simulink model "Traj_plt"  (R2023a)
settings: Solver=VariableStepAuto  StartTime=0.0  StopTime=inf  RelTol=1e-3
values from neighbouring files (symbols this model uses):
  beta = beta_i'.*task    [Compare1.m]    (also in Compare2.m; Final1.m; Final2.m; Final3.m)
undefined symbols (not defined in the file or in its folder): B_prev, Bst, Bst_prev, convertStringsToChars, dist_C, DroneMass, Earth, Gravity, h_ref, initialState, quad_pos, sinit, stack_size, task_mat, WGS84
libraries: slpidlib x66, aerolibconvert2 x11, aerolibtransform2 x11, uavalgslib x11, dspsrcs4 x1
(part 2 of 12)

== system Traj_plt/agent_4/Quad_1/Inner Loop and Plant Model ==
  PositionCmds : Inport
  Low-FidelityModel : Subsystem  VariantControl=plantModelFi ==0
  Out1 : Outport

== system Traj_plt/agent_5/Quad_1/Inner Loop and Plant Model ==
  PositionCmds : Inport
  Low-FidelityModel : Subsystem  VariantControl=plantModelFi ==0
  Out1 : Outport

== system Traj_plt/agent_6/Quad_1/Inner Loop and Plant Model ==
  PositionCmds : Inport
  Low-FidelityModel : Subsystem  VariantControl=plantModelFi ==0
  Out1 : Outport

== system Traj_plt/agent_7/Quad_1/Inner Loop and Plant Model ==
  PositionCmds : Inport
  Low-FidelityModel : Subsystem  VariantControl=plantModelFi ==0
  Out1 : Outport

== system Traj_plt/agent_8/Quad_1/Inner Loop and Plant Model ==
  PositionCmds : Inport
  Low-FidelityModel : Subsystem  VariantControl=plantModelFi ==0
  Out1 : Outport

== system Traj_plt/agent_9/Quad_1/Inner Loop and Plant Model ==
  PositionCmds : Inport
  Low-FidelityModel : Subsystem  VariantControl=plantModelFi ==0
  Out1 : Outport

== system Traj_plt/agent_1/Quad_1/Inner Loop and Plant Model/Low-FidelityModel ==
  PositionCmds : Inport
  Assemble UAV State Bus : Subsystem
  Bus Creator : BusCreator  Inputs=1
  Bus Creator1 : BusCreator  Inputs=1  OutDataTypeStr=Bus: uavGuidanceEnvironmentBus  NonVirtualBus=on
  Constant : Constant  Value=9.8  OutDataTypeStr=single
      settings: AttributesFormatString=%<Value>
  Position and Acceleration Control : Subsystem
  Quadrotor Plant : Subsystem  AncestorBlock=uavalgslib/Guidance Model  mask(Guidance Model){ModelType=MultirotorGuidance, SpecifiedDataType=single, SimulateUsing=Code generation, InitialWorldPositionMultirotor=quad_pos(:,1), InitialWorldVelocityMultirotor=[0; 0; 0], InitialEulerZYXMultirotor=[0; 0; 0], InitialBodyAngularRateRPYMultirotor=[0; 0; 0], InitialThrustMultirotor=0, InitialNorthFixedWing=0, InitialEastFixedWing=0, InitialHeightFixedWing=0, InitialAirSpeedFixedWing=0, InitialHeadingAngleFixedWing=0, InitialFlightPathAngleFixedWing=0, InitialRollAngleFixedWing=0, InitialRollAngleRateFixedWing=0, PDRollMultirotor=[3402.97,116.67], PDPitchMultirotor=[3402.97, 116.67], PYawRateMultirotor=1950, PThrustMultirotor=39, MassMultirotor=0.1, PHeightFixedWing=3.9, PHeadingAngleFixedWing=3.9, PFlightPathAngleFixedWing=39, PDRollFixedWing=[3402.97, 116.67], PAirSpeedFixedWing=1, FlightPathAngleLimitsFixedWing=[-pi/2, pi/2], StateBusName='uavGuidanceStateBus', ControlBusName='uavGuidanceControlBus', EnvironmentBusName='uavGuidanceEnvironmentBus', DataType=single}
      mask prompts: ModelType "uav:robotsluav:guidancemodelblock:ModelType"; SpecifiedDataType "uav:robotsluav:guidancemodelblock:DataType"; SimulateUsing "SystemBlock:MATLABSystem:SimulateUsing"; InitialWorldPositionMultirotor "uav:robotsluav:guidancemodelblock:WorldPosition"; InitialWorldVelocityMultirotor "uav:robotsluav:guidancemodelblock:WorldVelocity"; InitialEulerZYXMultirotor "uav:robotsluav:guidancemodelblock:EulerZYX"; InitialBodyAngularRateRPYMultirotor "uav:robotsluav:guidancemodelblock:BodyAngularRateRPY"; InitialThrustMultirotor "uav:robotsluav:guidancemodelblock:Thrust"; InitialNorthFixedWing "uav:robotsluav:guidancemodelblock:NorthPosition"; InitialEastFixedWing "uav:robotsluav:guidancemodelblock:EastPosition"; InitialHeightFixedWing "uav:robotsluav:guidancemodelblock:Height"; InitialAirSpeedFixedWing "uav:robotsluav:guidancemodelblock:AirSpeed"; InitialHeadingAngleFixedWing "uav:robotsluav:guidancemodelblock:HeadingAngle"; InitialFlightPathAngleFixedWing "uav:robotsluav:guidancemodelblock:FlightPathAngle"; InitialRollAngleFixedWing "uav:robotsluav:guidancemodelblock:RollAngle"; InitialRollAngleRateFixedWing "uav:robotsluav:guidancemodelblock:RollAngleRate"; PDRollMultirotor "uav:robotsluav:guidancemodelblock:PDRoll"; PDPitchMultirotor "uav:robotsluav:guidancemodelblock:PDPitch"; PYawRateMultirotor "uav:robotsluav:guidancemodelblock:PYawRate"; PThrustMultirotor "uav:robotsluav:guidancemodelblock:PThrust"; MassMultirotor "uav:robotsluav:guidancemodelblock:Mass"; PHeightFixedWing "uav:robotsluav:guidancemodelblock:PHeight"; PHeadingAngleFixedWing "uav:robotsluav:guidancemodelblock:PHeadingAngle"; PFlightPathAngleFixedWing "uav:robotsluav:guidancemodelblock:PFlightPathAngle"; PDRollFixedWing "uav:robotsluav:guidancemodelblock:PDRollAngle"; PAirSpeedFixedWing "uav:robotsluav:guidancemodelblock:PAirSpeed"; FlightPathAngleLimitsFixedWing "uav:robotsluav:guidancemodelblock:MinMaxFlightPathAngle"; StateBusName "uav:robotsluav:guidancemodelblock:StateBusName"; ControlBusName "uav:robotsluav:guidancemodelblock:ControlBusName"; EnvironmentBusName "uav:robotsluav:guidancemodelblock:EnvironmentBusName"; DataType "uav:robotsluav:guidancemodelblock:ResolvedDataType"
      mask help: uav:robotsluav:guidancemodelblock:Description
      mask init:
      | ModelName = gcb;
      | 
      | % Validate bus names
      | uav.sluav.internal.guidancemodel.mask.validateBusNames(gcb);
      | 
      | [stateDimension, initialState, UAVType, UAVDataType, UAVConfig] = ...
      |     uav.sluav.internal.guidancemodel.mask.initialize(ModelName, ModelType, gcb);
      mask Help: eval('helpview(fullfile(docroot, ''uav'', ''helptargets.map''), ''uavGuidanceModelBlock'')');
      mask TypeOptions ModelType: uav:robotsluav:guidancemodelblock:ModelTypeMultirotor | uav:robotsluav:guidancemodelblock:ModelTypeFixedWing
      mask Callback ModelType:
      | % Change mask dialog
      | uav.sluav.internal.guidancemodel.mask.modelTypeCallback(gcb);
      | 
      | % Create buses for the UAV block
      | uav.sluav.internal.guidancemodel.mask.createUAVBuses(gcb);
      mask Callback SpecifiedDataType:
      | if ~strcmp(get_param(gcb, 'SpecifiedDataType'), '<data type expression>')
      |     % Resolve input type
      |     uav.sluav.internal.guidancemodel.mask.dataTypeCallback(gcb);
      | 
      |     % Create buses for the UAV block
      |     uav.sluav.internal.guidancemodel.mask.createUAVBuses(gcb);
      | end
      mask TypeOptions SimulateUsing: ComputeDerivative/SimulateUsing | StateVector2Struct/SimulateUsing
      mask Callback StateBusName:
      | % Validate bus names
      | uav.sluav.internal.guidancemodel.mask.validateBusNames(gcb);
      | 
      | % Create buses for the UAV block
      | uav.sluav.internal.guidancemodel.mask.createUAVBuses(gcb);
      mask Callback ControlBusName:
      | % Validate bus names
      | uav.sluav.internal.guidancemodel.mask.validateBusNames(gcb);
      | 
      | % Create buses for the UAV block
      | uav.sluav.internal.guidancemodel.mask.createUAVBuses(gcb);
      mask Callback EnvironmentBusName:
      | % Validate bus names
      | uav.sluav.internal.guidancemodel.mask.validateBusNames(gcb);
      | 
      | % Create buses for the UAV block
      | uav.sluav.internal.guidancemodel.mask.createUAVBuses(gcb);
      mask DialogControl ModelType Prompt: Model Type:
      mask DialogControl SpecifiedDataType Prompt: Data Type:
      mask DialogControl SimulateUsing Prompt: Simulate using:
      mask DialogControl SimulateUsing Tooltip: SystemBlock:MATLABSystem:SimulateUsingDescription
      mask DialogControl InitialStateTab Prompt: uav:robotsluav:guidancemodelblock:InitialState
      mask DialogControl InitialWorldPositionMultirotor Prompt: World Position
      mask DialogControl InitialWorldVelocityMultirotor Prompt: World Velocity
      mask DialogControl InitialEulerZYXMultirotor Prompt: Euler Angles (ZYX)
      mask DialogControl InitialBodyAngularRateRPYMultirotor Prompt: Body Angular Rate
      mask DialogControl InitialThrustMultirotor Prompt: Thrust
      mask DialogControl InitialNorthFixedWing Prompt: North Position
      mask DialogControl InitialEastFixedWing Prompt: East Position
      mask DialogControl InitialHeightFixedWing Prompt: Height
      mask DialogControl InitialAirSpeedFixedWing Prompt: Air Speed
      mask DialogControl InitialHeadingAngleFixedWing Prompt: Heading Angle
      mask DialogControl InitialFlightPathAngleFixedWing Prompt: Flight Path Angle
      mask DialogControl InitialRollAngleFixedWing Prompt: Roll Angle
      mask DialogControl InitialRollAngleRateFixedWing Prompt: Roll Angular Velocity
      mask DialogControl ConfigurationTab Prompt: uav:robotsluav:guidancemodelblock:Configuration
      mask DialogControl PDRollMultirotor Prompt: PD Roll
      mask DialogControl PDPitchMultirotor Prompt: PD Pitch
      mask DialogControl PYawRateMultirotor Prompt: P YawRate
      mask DialogControl PThrustMultirotor Prompt: P Thrust
      mask DialogControl MassMultirotor Prompt: Mass
      mask DialogControl PHeightFixedWing Prompt: P Height
      mask DialogControl PHeadingAngleFixedWing Prompt: P Heading Angle
      mask DialogControl PFlightPathAngleFixedWing Prompt: P Flight Path Angle
      mask DialogControl PDRollFixedWing Prompt: PD Roll Angle
      mask DialogControl PAirSpeedFixedWing Prompt: P Air Speed
      mask DialogControl FlightPathAngleLimitsFixedWing Prompt: Min/Max Flight Path Angle
      mask DialogControl BusNameTab Prompt: uav:robotsluav:guidancemodelblock:InputOutputBusNames
      mask DialogControl StateBusName Prompt: State Bus Name
      mask DialogControl ControlBusName Prompt: Control Bus Name
      mask DialogControl EnvironmentBusName Prompt: Environment Bus Name
      mask DialogControl DataType Prompt: Resolved Data Type
      mask Display:
      | port_label('input', 1, 'Control')
      | port_label('input', 2, 'Environment')
      | port_label('output', 1, 'State')
  Rate Transition1 : RateTransition  OutPortSampleTime=UAVSampleTime
  Rate Transition2 : RateTransition  OutPortSampleTime=UAVSampleTime
  Out1 : Outport
  wires:
  Constant/1 -> Bus Creator1/1  "Gravity"
  Bus Creator1/1 -> Quadrotor Plant/2(Environment)
  Position and Acceleration Control/1(Control Signal) -> Rate Transition2/1
  Quadrotor Plant/1(State) -> Rate Transition1/1
  Rate Transition2/1 -> Quadrotor Plant/1(Control)
  PositionCmds/1 -> Position and Acceleration Control/2(PositionCmd)
  Rate Transition1/1 -> Position and Acceleration Control/1(QuadRotorState), Assemble UAV State Bus/1(State)
  Bus Creator/1 -> Out1/1
  Assemble UAV State Bus/1(UAVState) -> Bus Creator/1

== system Traj_plt/agent_10/Quad_1/Inner Loop and Plant Model/Low-FidelityModel ==
  PositionCmds : Inport
  Assemble UAV State Bus : Subsystem
  Bus Creator : BusCreator  Inputs=1
  Bus Creator1 : BusCreator  Inputs=1  OutDataTypeStr=Bus: uavGuidanceEnvironmentBus  NonVirtualBus=on
  Constant : Constant  Value=9.8  OutDataTypeStr=single
      settings: AttributesFormatString=%<Value>
  Position and Acceleration Control : Subsystem
  Quadrotor Plant : Subsystem  AncestorBlock=uavalgslib/Guidance Model  mask(Guidance Model){ModelType=MultirotorGuidance, SpecifiedDataType=single, SimulateUsing=Code generation, InitialWorldPositionMultirotor=quad_pos(:,10), InitialWorldVelocityMultirotor=[0; 0; 0], InitialEulerZYXMultirotor=[0; 0; 0], InitialBodyAngularRateRPYMultirotor=[0; 0; 0], InitialThrustMultirotor=0, InitialNorthFixedWing=0, InitialEastFixedWing=0, InitialHeightFixedWing=0, InitialAirSpeedFixedWing=0, InitialHeadingAngleFixedWing=0, InitialFlightPathAngleFixedWing=0, InitialRollAngleFixedWing=0, InitialRollAngleRateFixedWing=0, PDRollMultirotor=[3402.97,116.67], PDPitchMultirotor=[3402.97, 116.67], PYawRateMultirotor=1950, PThrustMultirotor=39, MassMultirotor=0.1, PHeightFixedWing=3.9, PHeadingAngleFixedWing=3.9, PFlightPathAngleFixedWing=39, PDRollFixedWing=[3402.97, 116.67], PAirSpeedFixedWing=1, FlightPathAngleLimitsFixedWing=[-pi/2, pi/2], StateBusName='uavGuidanceStateBus', ControlBusName='uavGuidanceControlBus', EnvironmentBusName='uavGuidanceEnvironmentBus', DataType=single}
      mask prompts: ModelType "uav:robotsluav:guidancemodelblock:ModelType"; SpecifiedDataType "uav:robotsluav:guidancemodelblock:DataType"; SimulateUsing "SystemBlock:MATLABSystem:SimulateUsing"; InitialWorldPositionMultirotor "uav:robotsluav:guidancemodelblock:WorldPosition"; InitialWorldVelocityMultirotor "uav:robotsluav:guidancemodelblock:WorldVelocity"; InitialEulerZYXMultirotor "uav:robotsluav:guidancemodelblock:EulerZYX"; InitialBodyAngularRateRPYMultirotor "uav:robotsluav:guidancemodelblock:BodyAngularRateRPY"; InitialThrustMultirotor "uav:robotsluav:guidancemodelblock:Thrust"; InitialNorthFixedWing "uav:robotsluav:guidancemodelblock:NorthPosition"; InitialEastFixedWing "uav:robotsluav:guidancemodelblock:EastPosition"; InitialHeightFixedWing "uav:robotsluav:guidancemodelblock:Height"; InitialAirSpeedFixedWing "uav:robotsluav:guidancemodelblock:AirSpeed"; InitialHeadingAngleFixedWing "uav:robotsluav:guidancemodelblock:HeadingAngle"; InitialFlightPathAngleFixedWing "uav:robotsluav:guidancemodelblock:FlightPathAngle"; InitialRollAngleFixedWing "uav:robotsluav:guidancemodelblock:RollAngle"; InitialRollAngleRateFixedWing "uav:robotsluav:guidancemodelblock:RollAngleRate"; PDRollMultirotor "uav:robotsluav:guidancemodelblock:PDRoll"; PDPitchMultirotor "uav:robotsluav:guidancemodelblock:PDPitch"; PYawRateMultirotor "uav:robotsluav:guidancemodelblock:PYawRate"; PThrustMultirotor "uav:robotsluav:guidancemodelblock:PThrust"; MassMultirotor "uav:robotsluav:guidancemodelblock:Mass"; PHeightFixedWing "uav:robotsluav:guidancemodelblock:PHeight"; PHeadingAngleFixedWing "uav:robotsluav:guidancemodelblock:PHeadingAngle"; PFlightPathAngleFixedWing "uav:robotsluav:guidancemodelblock:PFlightPathAngle"; PDRollFixedWing "uav:robotsluav:guidancemodelblock:PDRollAngle"; PAirSpeedFixedWing "uav:robotsluav:guidancemodelblock:PAirSpeed"; FlightPathAngleLimitsFixedWing "uav:robotsluav:guidancemodelblock:MinMaxFlightPathAngle"; StateBusName "uav:robotsluav:guidancemodelblock:StateBusName"; ControlBusName "uav:robotsluav:guidancemodelblock:ControlBusName"; EnvironmentBusName "uav:robotsluav:guidancemodelblock:EnvironmentBusName"; DataType "uav:robotsluav:guidancemodelblock:ResolvedDataType"
      mask help: uav:robotsluav:guidancemodelblock:Description
      mask init: same as Traj_plt/agent_1/Quad_1/Inner Loop and Plant Model/Low-FidelityModel/Quadrotor Plant
      mask Help: eval('helpview(fullfile(docroot, ''uav'', ''helptargets.map''), ''uavGuidanceModelBlock'')');
      mask TypeOptions ModelType: uav:robotsluav:guidancemodelblock:ModelTypeMultirotor | uav:robotsluav:guidancemodelblock:ModelTypeFixedWing
      mask Callback ModelType:
      | % Change mask dialog
      | uav.sluav.internal.guidancemodel.mask.modelTypeCallback(gcb);
      | 
      | % Create buses for the UAV block
      | uav.sluav.internal.guidancemodel.mask.createUAVBuses(gcb);
      mask Callback SpecifiedDataType:
      | if ~strcmp(get_param(gcb, 'SpecifiedDataType'), '<data type expression>')
      |     % Resolve input type
      |     uav.sluav.internal.guidancemodel.mask.dataTypeCallback(gcb);
      | 
      |     % Create buses for the UAV block
      |     uav.sluav.internal.guidancemodel.mask.createUAVBuses(gcb);
      | end
      mask TypeOptions SimulateUsing: ComputeDerivative/SimulateUsing | StateVector2Struct/SimulateUsing
      mask Callback StateBusName:
      | % Validate bus names
      | uav.sluav.internal.guidancemodel.mask.validateBusNames(gcb);
      | 
      | % Create buses for the UAV block
      | uav.sluav.internal.guidancemodel.mask.createUAVBuses(gcb);
      mask Callback ControlBusName:
      | % Validate bus names
      | uav.sluav.internal.guidancemodel.mask.validateBusNames(gcb);
      | 
      | % Create buses for the UAV block
      | uav.sluav.internal.guidancemodel.mask.createUAVBuses(gcb);
      mask Callback EnvironmentBusName:
      | % Validate bus names
      | uav.sluav.internal.guidancemodel.mask.validateBusNames(gcb);
      | 
      | % Create buses for the UAV block
      | uav.sluav.internal.guidancemodel.mask.createUAVBuses(gcb);
      mask DialogControl ModelType Prompt: Model Type:
      mask DialogControl SpecifiedDataType Prompt: Data Type:
      mask DialogControl SimulateUsing Prompt: Simulate using:
      mask DialogControl SimulateUsing Tooltip: SystemBlock:MATLABSystem:SimulateUsingDescription
      mask DialogControl InitialStateTab Prompt: uav:robotsluav:guidancemodelblock:InitialState
      mask DialogControl InitialWorldPositionMultirotor Prompt: World Position
      mask DialogControl InitialWorldVelocityMultirotor Prompt: World Velocity
      mask DialogControl InitialEulerZYXMultirotor Prompt: Euler Angles (ZYX)
      mask DialogControl InitialBodyAngularRateRPYMultirotor Prompt: Body Angular Rate
      mask DialogControl InitialThrustMultirotor Prompt: Thrust
      mask DialogControl InitialNorthFixedWing Prompt: North Position
      mask DialogControl InitialEastFixedWing Prompt: East Position
      mask DialogControl InitialHeightFixedWing Prompt: Height
      mask DialogControl InitialAirSpeedFixedWing Prompt: Air Speed
      mask DialogControl InitialHeadingAngleFixedWing Prompt: Heading Angle
      mask DialogControl InitialFlightPathAngleFixedWing Prompt: Flight Path Angle
      mask DialogControl InitialRollAngleFixedWing Prompt: Roll Angle
      mask DialogControl InitialRollAngleRateFixedWing Prompt: Roll Angular Velocity
      mask DialogControl ConfigurationTab Prompt: uav:robotsluav:guidancemodelblock:Configuration
      mask DialogControl PDRollMultirotor Prompt: PD Roll
      mask DialogControl PDPitchMultirotor Prompt: PD Pitch
      mask DialogControl PYawRateMultirotor Prompt: P YawRate
      mask DialogControl PThrustMultirotor Prompt: P Thrust
      mask DialogControl MassMultirotor Prompt: Mass
      mask DialogControl PHeightFixedWing Prompt: P Height
      mask DialogControl PHeadingAngleFixedWing Prompt: P Heading Angle
      mask DialogControl PFlightPathAngleFixedWing Prompt: P Flight Path Angle
      mask DialogControl PDRollFixedWing Prompt: PD Roll Angle
      mask DialogControl PAirSpeedFixedWing Prompt: P Air Speed
      mask DialogControl FlightPathAngleLimitsFixedWing Prompt: Min/Max Flight Path Angle
      mask DialogControl BusNameTab Prompt: uav:robotsluav:guidancemodelblock:InputOutputBusNames
      mask DialogControl StateBusName Prompt: State Bus Name
      mask DialogControl ControlBusName Prompt: Control Bus Name
      mask DialogControl EnvironmentBusName Prompt: Environment Bus Name
      mask DialogControl DataType Prompt: Resolved Data Type
      mask Display:
      | port_label('input', 1, 'Control')
      | port_label('input', 2, 'Environment')
      | port_label('output', 1, 'State')
  Rate Transition1 : RateTransition  OutPortSampleTime=UAVSampleTime
  Rate Transition2 : RateTransition  OutPortSampleTime=UAVSampleTime
  Out1 : Outport
  wires:
  Constant/1 -> Bus Creator1/1  "Gravity"
  Bus Creator1/1 -> Quadrotor Plant/2(Environment)
  Position and Acceleration Control/1(Control Signal) -> Rate Transition2/1
  Quadrotor Plant/1(State) -> Rate Transition1/1
  Rate Transition2/1 -> Quadrotor Plant/1(Control)
  PositionCmds/1 -> Position and Acceleration Control/2(PositionCmd)
  Rate Transition1/1 -> Position and Acceleration Control/1(QuadRotorState), Assemble UAV State Bus/1(State)
  Bus Creator/1 -> Out1/1
  Assemble UAV State Bus/1(UAVState) -> Bus Creator/1

== system Traj_plt/agent_11/Quad_1/Inner Loop and Plant Model/Low-FidelityModel ==
  PositionCmds : Inport
  Assemble UAV State Bus : Subsystem
  Bus Creator : BusCreator  Inputs=1
  Bus Creator1 : BusCreator  Inputs=1  OutDataTypeStr=Bus: uavGuidanceEnvironmentBus  NonVirtualBus=on
  Constant : Constant  Value=9.8  OutDataTypeStr=single
      settings: AttributesFormatString=%<Value>
  Position and Acceleration Control : Subsystem
  Quadrotor Plant : Subsystem  AncestorBlock=uavalgslib/Guidance Model  mask(Guidance Model){ModelType=MultirotorGuidance, SpecifiedDataType=single, SimulateUsing=Code generation, InitialWorldPositionMultirotor=quad_pos(:,6), InitialWorldVelocityMultirotor=[0; 0; 0], InitialEulerZYXMultirotor=[0; 0; 0], InitialBodyAngularRateRPYMultirotor=[0; 0; 0], InitialThrustMultirotor=0, InitialNorthFixedWing=0, InitialEastFixedWing=0, InitialHeightFixedWing=0, InitialAirSpeedFixedWing=0, InitialHeadingAngleFixedWing=0, InitialFlightPathAngleFixedWing=0, InitialRollAngleFixedWing=0, InitialRollAngleRateFixedWing=0, PDRollMultirotor=[3402.97,116.67], PDPitchMultirotor=[3402.97, 116.67], PYawRateMultirotor=1950, PThrustMultirotor=39, MassMultirotor=0.1, PHeightFixedWing=3.9, PHeadingAngleFixedWing=3.9, PFlightPathAngleFixedWing=39, PDRollFixedWing=[3402.97, 116.67], PAirSpeedFixedWing=1, FlightPathAngleLimitsFixedWing=[-pi/2, pi/2], StateBusName='uavGuidanceStateBus', ControlBusName='uavGuidanceControlBus', EnvironmentBusName='uavGuidanceEnvironmentBus', DataType=single}
      mask prompts: ModelType "uav:robotsluav:guidancemodelblock:ModelType"; SpecifiedDataType "uav:robotsluav:guidancemodelblock:DataType"; SimulateUsing "SystemBlock:MATLABSystem:SimulateUsing"; InitialWorldPositionMultirotor "uav:robotsluav:guidancemodelblock:WorldPosition"; InitialWorldVelocityMultirotor "uav:robotsluav:guidancemodelblock:WorldVelocity"; InitialEulerZYXMultirotor "uav:robotsluav:guidancemodelblock:EulerZYX"; InitialBodyAngularRateRPYMultirotor "uav:robotsluav:guidancemodelblock:BodyAngularRateRPY"; InitialThrustMultirotor "uav:robotsluav:guidancemodelblock:Thrust"; InitialNorthFixedWing "uav:robotsluav:guidancemodelblock:NorthPosition"; InitialEastFixedWing "uav:robotsluav:guidancemodelblock:EastPosition"; InitialHeightFixedWing "uav:robotsluav:guidancemodelblock:Height"; InitialAirSpeedFixedWing "uav:robotsluav:guidancemodelblock:AirSpeed"; InitialHeadingAngleFixedWing "uav:robotsluav:guidancemodelblock:HeadingAngle"; InitialFlightPathAngleFixedWing "uav:robotsluav:guidancemodelblock:FlightPathAngle"; InitialRollAngleFixedWing "uav:robotsluav:guidancemodelblock:RollAngle"; InitialRollAngleRateFixedWing "uav:robotsluav:guidancemodelblock:RollAngleRate"; PDRollMultirotor "uav:robotsluav:guidancemodelblock:PDRoll"; PDPitchMultirotor "uav:robotsluav:guidancemodelblock:PDPitch"; PYawRateMultirotor "uav:robotsluav:guidancemodelblock:PYawRate"; PThrustMultirotor "uav:robotsluav:guidancemodelblock:PThrust"; MassMultirotor "uav:robotsluav:guidancemodelblock:Mass"; PHeightFixedWing "uav:robotsluav:guidancemodelblock:PHeight"; PHeadingAngleFixedWing "uav:robotsluav:guidancemodelblock:PHeadingAngle"; PFlightPathAngleFixedWing "uav:robotsluav:guidancemodelblock:PFlightPathAngle"; PDRollFixedWing "uav:robotsluav:guidancemodelblock:PDRollAngle"; PAirSpeedFixedWing "uav:robotsluav:guidancemodelblock:PAirSpeed"; FlightPathAngleLimitsFixedWing "uav:robotsluav:guidancemodelblock:MinMaxFlightPathAngle"; StateBusName "uav:robotsluav:guidancemodelblock:StateBusName"; ControlBusName "uav:robotsluav:guidancemodelblock:ControlBusName"; EnvironmentBusName "uav:robotsluav:guidancemodelblock:EnvironmentBusName"; DataType "uav:robotsluav:guidancemodelblock:ResolvedDataType"
      mask help: uav:robotsluav:guidancemodelblock:Description
      mask init: same as Traj_plt/agent_1/Quad_1/Inner Loop and Plant Model/Low-FidelityModel/Quadrotor Plant
      mask Help: eval('helpview(fullfile(docroot, ''uav'', ''helptargets.map''), ''uavGuidanceModelBlock'')');
      mask TypeOptions ModelType: uav:robotsluav:guidancemodelblock:ModelTypeMultirotor | uav:robotsluav:guidancemodelblock:ModelTypeFixedWing
      mask Callback ModelType:
      | % Change mask dialog
      | uav.sluav.internal.guidancemodel.mask.modelTypeCallback(gcb);
      | 
      | % Create buses for the UAV block
      | uav.sluav.internal.guidancemodel.mask.createUAVBuses(gcb);
      mask Callback SpecifiedDataType:
      | if ~strcmp(get_param(gcb, 'SpecifiedDataType'), '<data type expression>')
      |     % Resolve input type
      |     uav.sluav.internal.guidancemodel.mask.dataTypeCallback(gcb);
      | 
      |     % Create buses for the UAV block
      |     uav.sluav.internal.guidancemodel.mask.createUAVBuses(gcb);
      | end
      mask TypeOptions SimulateUsing: ComputeDerivative/SimulateUsing | StateVector2Struct/SimulateUsing
      mask Callback StateBusName:
      | % Validate bus names
      | uav.sluav.internal.guidancemodel.mask.validateBusNames(gcb);
      | 
      | % Create buses for the UAV block
      | uav.sluav.internal.guidancemodel.mask.createUAVBuses(gcb);
      mask Callback ControlBusName:
      | % Validate bus names
      | uav.sluav.internal.guidancemodel.mask.validateBusNames(gcb);
      | 
      | % Create buses for the UAV block
      | uav.sluav.internal.guidancemodel.mask.createUAVBuses(gcb);
      mask Callback EnvironmentBusName:
      | % Validate bus names
      | uav.sluav.internal.guidancemodel.mask.validateBusNames(gcb);
      | 
      | % Create buses for the UAV block
      | uav.sluav.internal.guidancemodel.mask.createUAVBuses(gcb);
      mask DialogControl ModelType Prompt: Model Type:
      mask DialogControl SpecifiedDataType Prompt: Data Type:
      mask DialogControl SimulateUsing Prompt: Simulate using:
      mask DialogControl SimulateUsing Tooltip: SystemBlock:MATLABSystem:SimulateUsingDescription
      mask DialogControl InitialStateTab Prompt: uav:robotsluav:guidancemodelblock:InitialState
      mask DialogControl InitialWorldPositionMultirotor Prompt: World Position
      mask DialogControl InitialWorldVelocityMultirotor Prompt: World Velocity
      mask DialogControl InitialEulerZYXMultirotor Prompt: Euler Angles (ZYX)
      mask DialogControl InitialBodyAngularRateRPYMultirotor Prompt: Body Angular Rate
      mask DialogControl InitialThrustMultirotor Prompt: Thrust
      mask DialogControl InitialNorthFixedWing Prompt: North Position
      mask DialogControl InitialEastFixedWing Prompt: East Position
      mask DialogControl InitialHeightFixedWing Prompt: Height
      mask DialogControl InitialAirSpeedFixedWing Prompt: Air Speed
      mask DialogControl InitialHeadingAngleFixedWing Prompt: Heading Angle
      mask DialogControl InitialFlightPathAngleFixedWing Prompt: Flight Path Angle
      mask DialogControl InitialRollAngleFixedWing Prompt: Roll Angle
      mask DialogControl InitialRollAngleRateFixedWing Prompt: Roll Angular Velocity
      mask DialogControl ConfigurationTab Prompt: uav:robotsluav:guidancemodelblock:Configuration
      mask DialogControl PDRollMultirotor Prompt: PD Roll
      mask DialogControl PDPitchMultirotor Prompt: PD Pitch
      mask DialogControl PYawRateMultirotor Prompt: P YawRate
      mask DialogControl PThrustMultirotor Prompt: P Thrust
      mask DialogControl MassMultirotor Prompt: Mass
      mask DialogControl PHeightFixedWing Prompt: P Height
      mask DialogControl PHeadingAngleFixedWing Prompt: P Heading Angle
      mask DialogControl PFlightPathAngleFixedWing Prompt: P Flight Path Angle
      mask DialogControl PDRollFixedWing Prompt: PD Roll Angle
      mask DialogControl PAirSpeedFixedWing Prompt: P Air Speed
      mask DialogControl FlightPathAngleLimitsFixedWing Prompt: Min/Max Flight Path Angle
      mask DialogControl BusNameTab Prompt: uav:robotsluav:guidancemodelblock:InputOutputBusNames
      mask DialogControl StateBusName Prompt: State Bus Name
      mask DialogControl ControlBusName Prompt: Control Bus Name
      mask DialogControl EnvironmentBusName Prompt: Environment Bus Name
      mask DialogControl DataType Prompt: Resolved Data Type
      mask Display:
      | port_label('input', 1, 'Control')
      | port_label('input', 2, 'Environment')
      | port_label('output', 1, 'State')
  Rate Transition1 : RateTransition  OutPortSampleTime=UAVSampleTime
  Rate Transition2 : RateTransition  OutPortSampleTime=UAVSampleTime
  Out1 : Outport
  wires:
  Constant/1 -> Bus Creator1/1  "Gravity"
  Bus Creator1/1 -> Quadrotor Plant/2(Environment)
  Position and Acceleration Control/1(Control Signal) -> Rate Transition2/1
  Quadrotor Plant/1(State) -> Rate Transition1/1
  Rate Transition2/1 -> Quadrotor Plant/1(Control)
  PositionCmds/1 -> Position and Acceleration Control/2(PositionCmd)
  Rate Transition1/1 -> Position and Acceleration Control/1(QuadRotorState), Assemble UAV State Bus/1(State)
  Bus Creator/1 -> Out1/1
  Assemble UAV State Bus/1(UAVState) -> Bus Creator/1

== system Traj_plt/agent_2/Quad_1/Inner Loop and Plant Model/Low-FidelityModel ==
  PositionCmds : Inport
  Assemble UAV State Bus : Subsystem
  Bus Creator : BusCreator  Inputs=1
  Bus Creator1 : BusCreator  Inputs=1  OutDataTypeStr=Bus: uavGuidanceEnvironmentBus  NonVirtualBus=on
  Constant : Constant  Value=9.8  OutDataTypeStr=single
      settings: AttributesFormatString=%<Value>
  Position and Acceleration Control : Subsystem
  Quadrotor Plant : Subsystem  AncestorBlock=uavalgslib/Guidance Model  mask(Guidance Model){ModelType=MultirotorGuidance, SpecifiedDataType=single, SimulateUsing=Code generation, InitialWorldPositionMultirotor=quad_pos(:,2), InitialWorldVelocityMultirotor=[0; 0; 0], InitialEulerZYXMultirotor=[0; 0; 0], InitialBodyAngularRateRPYMultirotor=[0; 0; 0], InitialThrustMultirotor=0, InitialNorthFixedWing=0, InitialEastFixedWing=0, InitialHeightFixedWing=0, InitialAirSpeedFixedWing=0, InitialHeadingAngleFixedWing=0, InitialFlightPathAngleFixedWing=0, InitialRollAngleFixedWing=0, InitialRollAngleRateFixedWing=0, PDRollMultirotor=[3402.97,116.67], PDPitchMultirotor=[3402.97, 116.67], PYawRateMultirotor=1950, PThrustMultirotor=39, MassMultirotor=0.1, PHeightFixedWing=3.9, PHeadingAngleFixedWing=3.9, PFlightPathAngleFixedWing=39, PDRollFixedWing=[3402.97, 116.67], PAirSpeedFixedWing=1, FlightPathAngleLimitsFixedWing=[-pi/2, pi/2], StateBusName='uavGuidanceStateBus', ControlBusName='uavGuidanceControlBus', EnvironmentBusName='uavGuidanceEnvironmentBus', DataType=single}
      mask prompts: ModelType "uav:robotsluav:guidancemodelblock:ModelType"; SpecifiedDataType "uav:robotsluav:guidancemodelblock:DataType"; SimulateUsing "SystemBlock:MATLABSystem:SimulateUsing"; InitialWorldPositionMultirotor "uav:robotsluav:guidancemodelblock:WorldPosition"; InitialWorldVelocityMultirotor "uav:robotsluav:guidancemodelblock:WorldVelocity"; InitialEulerZYXMultirotor "uav:robotsluav:guidancemodelblock:EulerZYX"; InitialBodyAngularRateRPYMultirotor "uav:robotsluav:guidancemodelblock:BodyAngularRateRPY"; InitialThrustMultirotor "uav:robotsluav:guidancemodelblock:Thrust"; InitialNorthFixedWing "uav:robotsluav:guidancemodelblock:NorthPosition"; InitialEastFixedWing "uav:robotsluav:guidancemodelblock:EastPosition"; InitialHeightFixedWing "uav:robotsluav:guidancemodelblock:Height"; InitialAirSpeedFixedWing "uav:robotsluav:guidancemodelblock:AirSpeed"; InitialHeadingAngleFixedWing "uav:robotsluav:guidancemodelblock:HeadingAngle"; InitialFlightPathAngleFixedWing "uav:robotsluav:guidancemodelblock:FlightPathAngle"; InitialRollAngleFixedWing "uav:robotsluav:guidancemodelblock:RollAngle"; InitialRollAngleRateFixedWing "uav:robotsluav:guidancemodelblock:RollAngleRate"; PDRollMultirotor "uav:robotsluav:guidancemodelblock:PDRoll"; PDPitchMultirotor "uav:robotsluav:guidancemodelblock:PDPitch"; PYawRateMultirotor "uav:robotsluav:guidancemodelblock:PYawRate"; PThrustMultirotor "uav:robotsluav:guidancemodelblock:PThrust"; MassMultirotor "uav:robotsluav:guidancemodelblock:Mass"; PHeightFixedWing "uav:robotsluav:guidancemodelblock:PHeight"; PHeadingAngleFixedWing "uav:robotsluav:guidancemodelblock:PHeadingAngle"; PFlightPathAngleFixedWing "uav:robotsluav:guidancemodelblock:PFlightPathAngle"; PDRollFixedWing "uav:robotsluav:guidancemodelblock:PDRollAngle"; PAirSpeedFixedWing "uav:robotsluav:guidancemodelblock:PAirSpeed"; FlightPathAngleLimitsFixedWing "uav:robotsluav:guidancemodelblock:MinMaxFlightPathAngle"; StateBusName "uav:robotsluav:guidancemodelblock:StateBusName"; ControlBusName "uav:robotsluav:guidancemodelblock:ControlBusName"; EnvironmentBusName "uav:robotsluav:guidancemodelblock:EnvironmentBusName"; DataType "uav:robotsluav:guidancemodelblock:ResolvedDataType"
      mask help: uav:robotsluav:guidancemodelblock:Description
      mask init: same as Traj_plt/agent_1/Quad_1/Inner Loop and Plant Model/Low-FidelityModel/Quadrotor Plant
      mask Help: eval('helpview(fullfile(docroot, ''uav'', ''helptargets.map''), ''uavGuidanceModelBlock'')');
      mask TypeOptions ModelType: uav:robotsluav:guidancemodelblock:ModelTypeMultirotor | uav:robotsluav:guidancemodelblock:ModelTypeFixedWing
      mask Callback ModelType:
      | % Change mask dialog
      | uav.sluav.internal.guidancemodel.mask.modelTypeCallback(gcb);
      | 
      | % Create buses for the UAV block
      | uav.sluav.internal.guidancemodel.mask.createUAVBuses(gcb);
      mask Callback SpecifiedDataType:
      | if ~strcmp(get_param(gcb, 'SpecifiedDataType'), '<data type expression>')
      |     % Resolve input type
      |     uav.sluav.internal.guidancemodel.mask.dataTypeCallback(gcb);
      | 
      |     % Create buses for the UAV block
      |     uav.sluav.internal.guidancemodel.mask.createUAVBuses(gcb);
      | end
      mask TypeOptions SimulateUsing: ComputeDerivative/SimulateUsing | StateVector2Struct/SimulateUsing
      mask Callback StateBusName:
      | % Validate bus names
      | uav.sluav.internal.guidancemodel.mask.validateBusNames(gcb);
      | 
      | % Create buses for the UAV block
      | uav.sluav.internal.guidancemodel.mask.createUAVBuses(gcb);
      mask Callback ControlBusName:
      | % Validate bus names
      | uav.sluav.internal.guidancemodel.mask.validateBusNames(gcb);
      | 
      | % Create buses for the UAV block
      | uav.sluav.internal.guidancemodel.mask.createUAVBuses(gcb);
      mask Callback EnvironmentBusName:
      | % Validate bus names
      | uav.sluav.internal.guidancemodel.mask.validateBusNames(gcb);
      | 
      | % Create buses for the UAV block
      | uav.sluav.internal.guidancemodel.mask.createUAVBuses(gcb);
      mask DialogControl ModelType Prompt: Model Type:
      mask DialogControl SpecifiedDataType Prompt: Data Type:
      mask DialogControl SimulateUsing Prompt: Simulate using:
      mask DialogControl SimulateUsing Tooltip: SystemBlock:MATLABSystem:SimulateUsingDescription
      mask DialogControl InitialStateTab Prompt: uav:robotsluav:guidancemodelblock:InitialState
      mask DialogControl InitialWorldPositionMultirotor Prompt: World Position
      mask DialogControl InitialWorldVelocityMultirotor Prompt: World Velocity
      mask DialogControl InitialEulerZYXMultirotor Prompt: Euler Angles (ZYX)
      mask DialogControl InitialBodyAngularRateRPYMultirotor Prompt: Body Angular Rate
      mask DialogControl InitialThrustMultirotor Prompt: Thrust
      mask DialogControl InitialNorthFixedWing Prompt: North Position
      mask DialogControl InitialEastFixedWing Prompt: East Position
      mask DialogControl InitialHeightFixedWing Prompt: Height
      mask DialogControl InitialAirSpeedFixedWing Prompt: Air Speed
      mask DialogControl InitialHeadingAngleFixedWing Prompt: Heading Angle
      mask DialogControl InitialFlightPathAngleFixedWing Prompt: Flight Path Angle
      mask DialogControl InitialRollAngleFixedWing Prompt: Roll Angle
      mask DialogControl InitialRollAngleRateFixedWing Prompt: Roll Angular Velocity
      mask DialogControl ConfigurationTab Prompt: uav:robotsluav:guidancemodelblock:Configuration
      mask DialogControl PDRollMultirotor Prompt: PD Roll
      mask DialogControl PDPitchMultirotor Prompt: PD Pitch
      mask DialogControl PYawRateMultirotor Prompt: P YawRate
      mask DialogControl PThrustMultirotor Prompt: P Thrust
      mask DialogControl MassMultirotor Prompt: Mass
      mask DialogControl PHeightFixedWing Prompt: P Height
      mask DialogControl PHeadingAngleFixedWing Prompt: P Heading Angle
      mask DialogControl PFlightPathAngleFixedWing Prompt: P Flight Path Angle
      mask DialogControl PDRollFixedWing Prompt: PD Roll Angle
      mask DialogControl PAirSpeedFixedWing Prompt: P Air Speed
      mask DialogControl FlightPathAngleLimitsFixedWing Prompt: Min/Max Flight Path Angle
      mask DialogControl BusNameTab Prompt: uav:robotsluav:guidancemodelblock:InputOutputBusNames
      mask DialogControl StateBusName Prompt: State Bus Name
      mask DialogControl ControlBusName Prompt: Control Bus Name
      mask DialogControl EnvironmentBusName Prompt: Environment Bus Name
      mask DialogControl DataType Prompt: Resolved Data Type
      mask Display:
      | port_label('input', 1, 'Control')
      | port_label('input', 2, 'Environment')
      | port_label('output', 1, 'State')
  Rate Transition1 : RateTransition  OutPortSampleTime=UAVSampleTime
  Rate Transition2 : RateTransition  OutPortSampleTime=UAVSampleTime
  Out1 : Outport
  wires:
  Constant/1 -> Bus Creator1/1  "Gravity"
  Bus Creator1/1 -> Quadrotor Plant/2(Environment)
  Position and Acceleration Control/1(Control Signal) -> Rate Transition2/1
  Quadrotor Plant/1(State) -> Rate Transition1/1
  Rate Transition2/1 -> Quadrotor Plant/1(Control)
  PositionCmds/1 -> Position and Acceleration Control/2(PositionCmd)
  Rate Transition1/1 -> Position and Acceleration Control/1(QuadRotorState), Assemble UAV State Bus/1(State)
  Bus Creator/1 -> Out1/1
  Assemble UAV State Bus/1(UAVState) -> Bus Creator/1

== system Traj_plt/agent_3/Quad_1/Inner Loop and Plant Model/Low-FidelityModel ==
  PositionCmds : Inport
  Assemble UAV State Bus : Subsystem
  Bus Creator : BusCreator  Inputs=1
  Bus Creator1 : BusCreator  Inputs=1  OutDataTypeStr=Bus: uavGuidanceEnvironmentBus  NonVirtualBus=on
  Constant : Constant  Value=9.8  OutDataTypeStr=single
      settings: AttributesFormatString=%<Value>
  Position and Acceleration Control : Subsystem
  Quadrotor Plant : Subsystem  AncestorBlock=uavalgslib/Guidance Model  mask(Guidance Model){ModelType=MultirotorGuidance, SpecifiedDataType=single, SimulateUsing=Code generation, InitialWorldPositionMultirotor=quad_pos(:,3), InitialWorldVelocityMultirotor=[0; 0; 0], InitialEulerZYXMultirotor=[0; 0; 0], InitialBodyAngularRateRPYMultirotor=[0; 0; 0], InitialThrustMultirotor=0, InitialNorthFixedWing=0, InitialEastFixedWing=0, InitialHeightFixedWing=0, InitialAirSpeedFixedWing=0, InitialHeadingAngleFixedWing=0, InitialFlightPathAngleFixedWing=0, InitialRollAngleFixedWing=0, InitialRollAngleRateFixedWing=0, PDRollMultirotor=[3402.97,116.67], PDPitchMultirotor=[3402.97, 116.67], PYawRateMultirotor=1950, PThrustMultirotor=39, MassMultirotor=0.1, PHeightFixedWing=3.9, PHeadingAngleFixedWing=3.9, PFlightPathAngleFixedWing=39, PDRollFixedWing=[3402.97, 116.67], PAirSpeedFixedWing=1, FlightPathAngleLimitsFixedWing=[-pi/2, pi/2], StateBusName='uavGuidanceStateBus', ControlBusName='uavGuidanceControlBus', EnvironmentBusName='uavGuidanceEnvironmentBus', DataType=single}
      mask prompts: ModelType "uav:robotsluav:guidancemodelblock:ModelType"; SpecifiedDataType "uav:robotsluav:guidancemodelblock:DataType"; SimulateUsing "SystemBlock:MATLABSystem:SimulateUsing"; InitialWorldPositionMultirotor "uav:robotsluav:guidancemodelblock:WorldPosition"; InitialWorldVelocityMultirotor "uav:robotsluav:guidancemodelblock:WorldVelocity"; InitialEulerZYXMultirotor "uav:robotsluav:guidancemodelblock:EulerZYX"; InitialBodyAngularRateRPYMultirotor "uav:robotsluav:guidancemodelblock:BodyAngularRateRPY"; InitialThrustMultirotor "uav:robotsluav:guidancemodelblock:Thrust"; InitialNorthFixedWing "uav:robotsluav:guidancemodelblock:NorthPosition"; InitialEastFixedWing "uav:robotsluav:guidancemodelblock:EastPosition"; InitialHeightFixedWing "uav:robotsluav:guidancemodelblock:Height"; InitialAirSpeedFixedWing "uav:robotsluav:guidancemodelblock:AirSpeed"; InitialHeadingAngleFixedWing "uav:robotsluav:guidancemodelblock:HeadingAngle"; InitialFlightPathAngleFixedWing "uav:robotsluav:guidancemodelblock:FlightPathAngle"; InitialRollAngleFixedWing "uav:robotsluav:guidancemodelblock:RollAngle"; InitialRollAngleRateFixedWing "uav:robotsluav:guidancemodelblock:RollAngleRate"; PDRollMultirotor "uav:robotsluav:guidancemodelblock:PDRoll"; PDPitchMultirotor "uav:robotsluav:guidancemodelblock:PDPitch"; PYawRateMultirotor "uav:robotsluav:guidancemodelblock:PYawRate"; PThrustMultirotor "uav:robotsluav:guidancemodelblock:PThrust"; MassMultirotor "uav:robotsluav:guidancemodelblock:Mass"; PHeightFixedWing "uav:robotsluav:guidancemodelblock:PHeight"; PHeadingAngleFixedWing "uav:robotsluav:guidancemodelblock:PHeadingAngle"; PFlightPathAngleFixedWing "uav:robotsluav:guidancemodelblock:PFlightPathAngle"; PDRollFixedWing "uav:robotsluav:guidancemodelblock:PDRollAngle"; PAirSpeedFixedWing "uav:robotsluav:guidancemodelblock:PAirSpeed"; FlightPathAngleLimitsFixedWing "uav:robotsluav:guidancemodelblock:MinMaxFlightPathAngle"; StateBusName "uav:robotsluav:guidancemodelblock:StateBusName"; ControlBusName "uav:robotsluav:guidancemodelblock:ControlBusName"; EnvironmentBusName "uav:robotsluav:guidancemodelblock:EnvironmentBusName"; DataType "uav:robotsluav:guidancemodelblock:ResolvedDataType"
      mask help: uav:robotsluav:guidancemodelblock:Description
      mask init: same as Traj_plt/agent_1/Quad_1/Inner Loop and Plant Model/Low-FidelityModel/Quadrotor Plant
      mask Help: eval('helpview(fullfile(docroot, ''uav'', ''helptargets.map''), ''uavGuidanceModelBlock'')');
      mask TypeOptions ModelType: uav:robotsluav:guidancemodelblock:ModelTypeMultirotor | uav:robotsluav:guidancemodelblock:ModelTypeFixedWing
      mask Callback ModelType:
      | % Change mask dialog
      | uav.sluav.internal.guidancemodel.mask.modelTypeCallback(gcb);
      | 
      | % Create buses for the UAV block
      | uav.sluav.internal.guidancemodel.mask.createUAVBuses(gcb);
      mask Callback SpecifiedDataType:
      | if ~strcmp(get_param(gcb, 'SpecifiedDataType'), '<data type expression>')
      |     % Resolve input type
      |     uav.sluav.internal.guidancemodel.mask.dataTypeCallback(gcb);
      | 
      |     % Create buses for the UAV block
      |     uav.sluav.internal.guidancemodel.mask.createUAVBuses(gcb);
      | end
      mask TypeOptions SimulateUsing: ComputeDerivative/SimulateUsing | StateVector2Struct/SimulateUsing
      mask Callback StateBusName:
      | % Validate bus names
      | uav.sluav.internal.guidancemodel.mask.validateBusNames(gcb);
      | 
      | % Create buses for the UAV block
      | uav.sluav.internal.guidancemodel.mask.createUAVBuses(gcb);
      mask Callback ControlBusName:
      | % Validate bus names
      | uav.sluav.internal.guidancemodel.mask.validateBusNames(gcb);
      | 
      | % Create buses for the UAV block
      | uav.sluav.internal.guidancemodel.mask.createUAVBuses(gcb);
      mask Callback EnvironmentBusName:
      | % Validate bus names
      | uav.sluav.internal.guidancemodel.mask.validateBusNames(gcb);
      | 
      | % Create buses for the UAV block
      | uav.sluav.internal.guidancemodel.mask.createUAVBuses(gcb);
      mask DialogControl ModelType Prompt: Model Type:
      mask DialogControl SpecifiedDataType Prompt: Data Type:
      mask DialogControl SimulateUsing Prompt: Simulate using:
      mask DialogControl SimulateUsing Tooltip: SystemBlock:MATLABSystem:SimulateUsingDescription
      mask DialogControl InitialStateTab Prompt: uav:robotsluav:guidancemodelblock:InitialState
      mask DialogControl InitialWorldPositionMultirotor Prompt: World Position
      mask DialogControl InitialWorldVelocityMultirotor Prompt: World Velocity
      mask DialogControl InitialEulerZYXMultirotor Prompt: Euler Angles (ZYX)
      mask DialogControl InitialBodyAngularRateRPYMultirotor Prompt: Body Angular Rate
      mask DialogControl InitialThrustMultirotor Prompt: Thrust
      mask DialogControl InitialNorthFixedWing Prompt: North Position
      mask DialogControl InitialEastFixedWing Prompt: East Position
      mask DialogControl InitialHeightFixedWing Prompt: Height
      mask DialogControl InitialAirSpeedFixedWing Prompt: Air Speed
      mask DialogControl InitialHeadingAngleFixedWing Prompt: Heading Angle
      mask DialogControl InitialFlightPathAngleFixedWing Prompt: Flight Path Angle
      mask DialogControl InitialRollAngleFixedWing Prompt: Roll Angle
      mask DialogControl InitialRollAngleRateFixedWing Prompt: Roll Angular Velocity
      mask DialogControl ConfigurationTab Prompt: uav:robotsluav:guidancemodelblock:Configuration
      mask DialogControl PDRollMultirotor Prompt: PD Roll
      mask DialogControl PDPitchMultirotor Prompt: PD Pitch
      mask DialogControl PYawRateMultirotor Prompt: P YawRate
      mask DialogControl PThrustMultirotor Prompt: P Thrust
      mask DialogControl MassMultirotor Prompt: Mass
      mask DialogControl PHeightFixedWing Prompt: P Height
      mask DialogControl PHeadingAngleFixedWing Prompt: P Heading Angle
      mask DialogControl PFlightPathAngleFixedWing Prompt: P Flight Path Angle
      mask DialogControl PDRollFixedWing Prompt: PD Roll Angle
      mask DialogControl PAirSpeedFixedWing Prompt: P Air Speed
      mask DialogControl FlightPathAngleLimitsFixedWing Prompt: Min/Max Flight Path Angle
      mask DialogControl BusNameTab Prompt: uav:robotsluav:guidancemodelblock:InputOutputBusNames
      mask DialogControl StateBusName Prompt: State Bus Name
      mask DialogControl ControlBusName Prompt: Control Bus Name
      mask DialogControl EnvironmentBusName Prompt: Environment Bus Name
      mask DialogControl DataType Prompt: Resolved Data Type
      mask Display:
      | port_label('input', 1, 'Control')
      | port_label('input', 2, 'Environment')
      | port_label('output', 1, 'State')
  Rate Transition1 : RateTransition  OutPortSampleTime=UAVSampleTime
  Rate Transition2 : RateTransition  OutPortSampleTime=UAVSampleTime
  Out1 : Outport
  wires:
  Constant/1 -> Bus Creator1/1  "Gravity"
  Bus Creator1/1 -> Quadrotor Plant/2(Environment)
  Position and Acceleration Control/1(Control Signal) -> Rate Transition2/1
  Quadrotor Plant/1(State) -> Rate Transition1/1
  Rate Transition2/1 -> Quadrotor Plant/1(Control)
  PositionCmds/1 -> Position and Acceleration Control/2(PositionCmd)
  Rate Transition1/1 -> Position and Acceleration Control/1(QuadRotorState), Assemble UAV State Bus/1(State)
  Bus Creator/1 -> Out1/1
  Assemble UAV State Bus/1(UAVState) -> Bus Creator/1
